simulink model "servo_control"  (R2024a)
settings: Solver=FixedStepAuto  StartTime=0.0  StopTime=inf  FixedStep=0.005  RelTol=1e-3  EnableMultiTasking=on
libraries: arduinolib x7
settings Model: ExtModeTrigDuration=2  Creator=ibrahim elshami  LastModifiedBy=ibrahim elshami
settings SolverCC: AutoInsertRateTranBlk=on
settings OptimizationCC: EnhancedBackFolding=on  PassReuseOutputArgsAs=Individual arguments  ZeroExternalMemoryAtStartup=off  ZeroInternalMemoryAtStartup=off  MaxStackSize=64  OptimizeBlockOrder=speed  DifferentSizesBufferReuse=on  OptimizationCustomize=off  EfficientTunableParamExpr=on
settings DebuggingCC: ParameterTunabilityLossMsg=error
settings HardwareCC: ProdBitPerPointer=32  ProdBitPerSizeT=32  ProdBitPerPtrDiffT=32  ProdLargestAtomicInteger=Long  ProdLargestAtomicFloat=Double  ProdWordSize=32  ProdHWDeviceType=ARM Compatible->ARM Cortex
settings SFSimCC: MATLABDynamicMemAlloc=off
settings RTWCC: Description=Embedded Coder  SystemTargetFile=ert.tlc  HardwareBoard=ESP32-WROOM(Arduino Compatible)  TLCOptions="-aInlineSetEventsForThisBaseRateFcn=TLC_FALSE -aSuppressMultiTaskScheduler=TLC_FALSE  -aRateBasedStepFcn=0"  TemplateMakefile=ert_default_tmf  Toolchain=ESP32  BuildConfiguration=Faster Runs
settings CodeAppCC: ForceParamTrailComments=on  IgnoreCustomStorageClasses=off  OperatorAnnotations=on  SimulinkDataObjDesc=on  SFDataObjDesc=on  InsertBlockDesc=on
settings ERTTargetCC: SupportContinuousTime=on  SupportVariableSizeSignals=on  ExtModeTransport=3  ExtModeStaticAlloc=on  ExtModeAutomaticAllocSize=off  ExtModeStaticAllocSize=65536  ExtModeMexFile=ext_xcp  ExtModeIntrfLevel=Level2 - Open

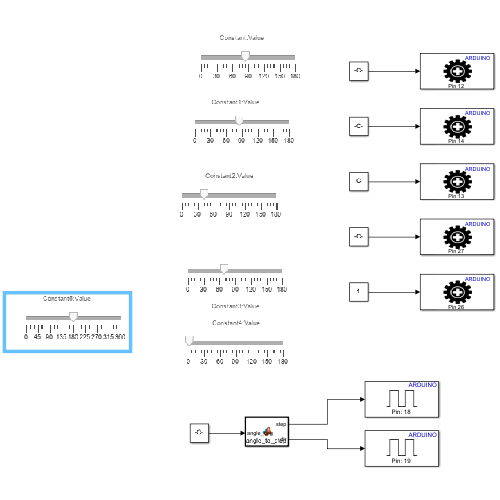
[thumbnail: Simulink's stored preview of the top-level diagram]
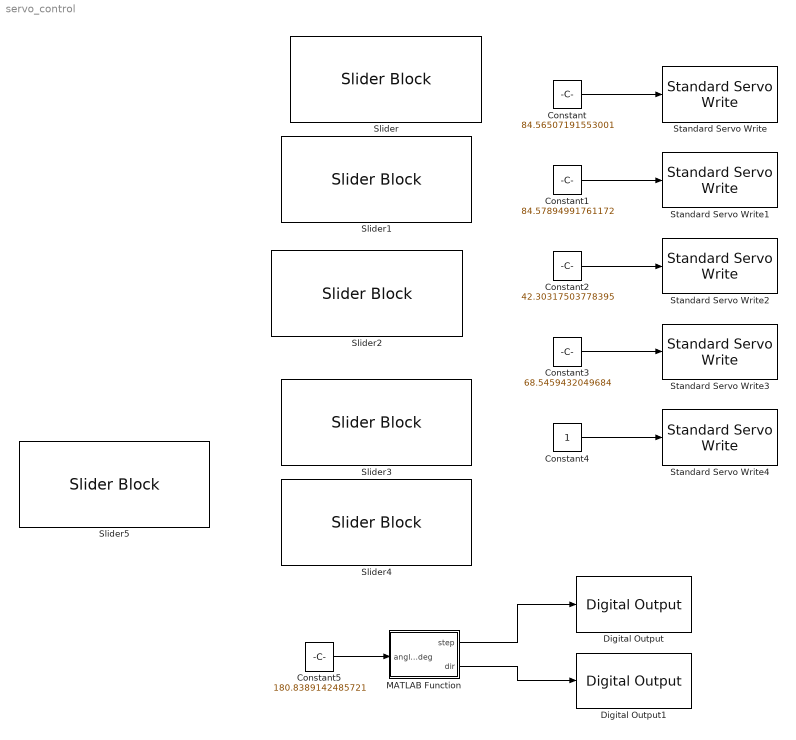
== system servo_control ==
  Constant : Constant  Value=84.56507191553001
  Constant1 : Constant  Value=84.57894991761172
  Constant2 : Constant  Value=42.30317503778395
  Constant3 : Constant  Value=68.5459432049684
  Constant4 : Constant
  Constant5 : Constant  Value=180.8389142485721
  Digital Output : arduinolib/Digital Output  pinNumber=18  Direction=output  blockPlatform=arduino
  Digital Output1 : arduinolib/Digital Output  pinNumber=19  Direction=output  blockPlatform=arduino
  MATLAB Function : MATLAB Function  TreatAsAtomicUnit=on
  Slider{,1..2,4} (4 alike) : SliderBlock  ScaleMax=180
  Slider3 : SliderBlock  LabelPosition=Bottom  ScaleMax=180
  Slider5 : SliderBlock  ScaleMax=360
  Standard Servo Write : arduinolib/Standard Servo Write  pinNumber=12  ServoIndex=0  blockPlatform=ARDUINO
  Standard Servo Write1 : arduinolib/Standard Servo Write  pinNumber=14  ServoIndex=1  blockPlatform=ARDUINO
  Standard Servo Write2 : arduinolib/Standard Servo Write  pinNumber=13  ServoIndex=2  blockPlatform=ARDUINO
  Standard Servo Write3 : arduinolib/Standard Servo Write  pinNumber=27  ServoIndex=3  blockPlatform=ARDUINO
  Standard Servo Write4 : arduinolib/Standard Servo Write  pinNumber=26  ServoIndex=4  blockPlatform=ARDUINO
  wires:
  Constant/1 -> Standard Servo Write/1
  Constant1/1 -> Standard Servo Write1/1
  Constant2/1 -> Standard Servo Write2/1
  Constant3/1 -> Standard Servo Write3/1
  Constant4/1 -> Standard Servo Write4/1
  Constant5/1 -> MATLAB Function/1(angle_deg)
  MATLAB Function/1(step) -> Digital Output/1
  MATLAB Function/2(dir) -> Digital Output1/1

== matlab function servo_control/MATLAB Function ==
  data: angle_deg input; step output; dir output
function [step, dir] = angle_to_step(angle_deg)
%#codegen

% ── Motor parameters ──────────────────────────────────
STEPS_PER_REV = 200;    % steps per full revolution
% Solver fixed step size must equal HALF_PERIOD
% e.g. 5000 us = 0.005 s  →  set solver step = 0.005

% ── Persistent state ──────────────────────────────────
persistent count target last_angle pulse_phase
if isempty(count)
    count       = int32(0);
    target      = int32(0);
    last_angle  = 0;
    pulse_phase = false;   % false = HIGH phase, true = LOW phase
end

% ── Direction ─────────────────────────────────────────
dir = angle_deg >= 0;

% ── Load new target when angle input changes ──────────
if angle_deg ~= last_angle
    target      = int32(round(abs(angle_deg) * STEPS_PER_REV / 360));
    count       = int32(0);
    last_angle  = angle_deg;
    pulse_phase = false;
end

% ── Two-phase pulse generation ────────────────────────
if count < target
    if ~pulse_phase
        % Phase 1: drive STEP HIGH for one solver tick (5000 us)
        step        = true;
        pulse_phase = true;    % next tick → go LOW
    else
        % Phase 2: drive STEP LOW for one solver tick (5000 us)
        step        = false;
        pulse_phase = false;   % next tick → next step
        count       = count + int32(1);   % count AFTER full pulse
    end
else
    step        = false;
    pulse_phase = false;
end
